simulink model "control_system"  (R2023a)
settings: Solver=VariableStepAuto  StartTime=0.0  StopTime=10.0  RelTol=1e-3
model workspace (MAT data in the model file):
  C_L = Simulink.Parameter
  C_L.Value = 1
  C_L.DataType = 'auto'
  C_L.Complexity = 'real'
  C_L.Dimensions = [1 1]
  C_R = Simulink.Parameter
  C_R.Value = 2
  C_R.DataType = 'auto'
  C_R.Complexity = 'real'
  C_R.Dimensions = [1 1]
  V = Simulink.Parameter
  V.Value = 1
  V.DataType = 'auto'
  V.DocUnits = 'm/s'
  V.Complexity = 'real'
  V.Dimensions = [1 1]
  b_w = Simulink.Parameter
  b_w.Value = 15
  b_w.DataType = 'auto'
  b_w.DocUnits = 'mm'
  b_w.Complexity = 'real'
  b_w.Dimensions = [1 1]
undefined symbols (not defined in the file): Ka
libraries: slpidlib x3
settings Model: Creator=gabrielle  LastModifiedBy=gabrielle

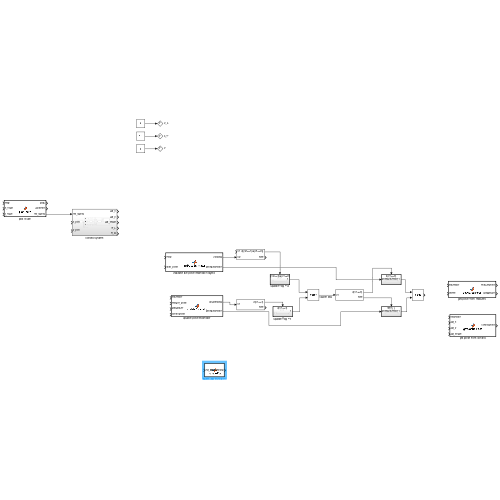
[thumbnail: Simulink's stored preview of the top-level diagram]
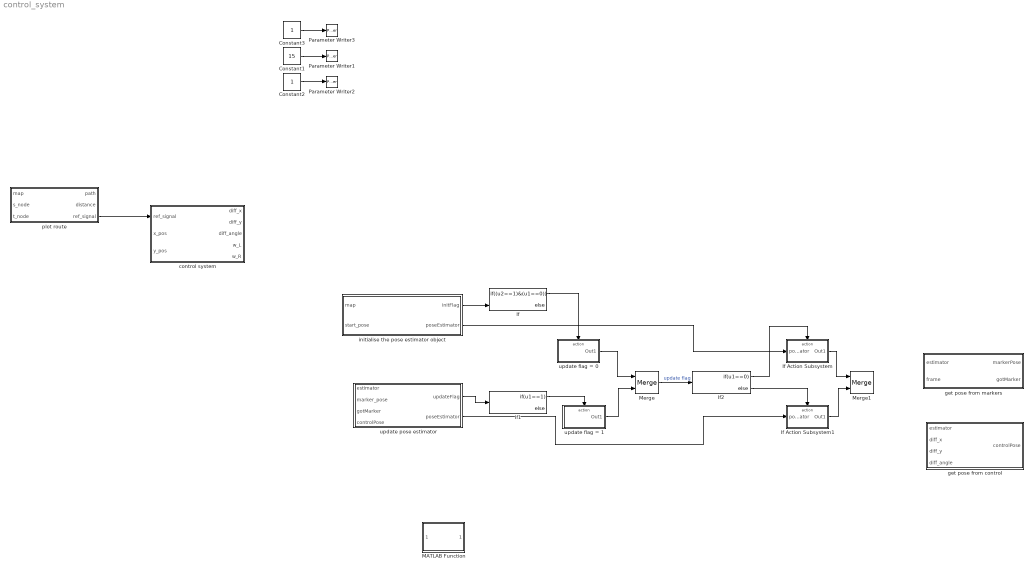
== system control_system ==
  Constant1 : Constant  Value=15
  Constant2 : Constant
  Constant3 : Constant
  If : If  NumInputs=2  IfExpression=(u2==1)&(u1==0)
  If Action Subsystem : Subsystem  TreatAsAtomicUnit=on
  If Action Subsystem1 : Subsystem  TreatAsAtomicUnit=on
  If1 : If  IfExpression=u1==1
  If2 : If  IfExpression=u1==0
  MATLAB Function : MATLAB Function  TreatAsAtomicUnit=on
  Merge : Merge  InitialOutput=0
  Merge1 : Merge  InitialOutput=0
  Parameter Writer1 : ParameterWriter  AccessWorkspaceVariable=on  WorkspaceVariableName=b_w
  Parameter Writer2 : ParameterWriter  AccessWorkspaceVariable=on  WorkspaceVariableName=V
  Parameter Writer3 : ParameterWriter  AccessWorkspaceVariable=on  WorkspaceVariableName=C_L
  control system : Subsystem
  get pose from control : MATLAB Function  TreatAsAtomicUnit=on
  get pose from markers : MATLAB Function  TreatAsAtomicUnit=on
  initialise the pose estimator object : MATLAB Function  TreatAsAtomicUnit=on
  plot route : MATLAB Function  TreatAsAtomicUnit=on
  update flag = 0 : Subsystem  TreatAsAtomicUnit=on
  update flag = 1 : Subsystem  TreatAsAtomicUnit=on
  update pose estimator : MATLAB Function  TreatAsAtomicUnit=on
  wires:
  Constant3/1 -> Parameter Writer3/1
  Constant1/1 -> Parameter Writer1/1
  Constant2/1 -> Parameter Writer2/1
  plot route/3(ref_signal) -> control system/1(ref_signal)
  initialise the pose estimator object/1(initFlag) -> If/2
  update pose estimator/1(updateFlag) -> If1/1
  update flag = 0/1(Out1) -> Merge/1
  update flag = 1/1(Out1) -> Merge/2
  If/1 -> update flag = 0/Action
  Merge/1 -> If2/1  "update flag"
  If1/1 -> update flag = 1/Action
  If2/1 -> If Action Subsystem/Action
  If2/2 -> If Action Subsystem1/Action
  initialise the pose estimator object/2(poseEstimator) -> If Action Subsystem/1(poseEstimator)
  update pose estimator/2(poseEstimator) -> If Action Subsystem1/1(poseEstimator)
  If Action Subsystem/1(Out1) -> Merge1/1
  If Action Subsystem1/1(Out1) -> Merge1/2

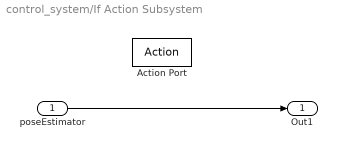
== system control_system/If Action Subsystem ==
  poseEstimator : Inport
  Action Port : ActionPort  ActionPortLabel=if(u1==0)
  Out1 : Outport
  wires:
  poseEstimator/1 -> Out1/1

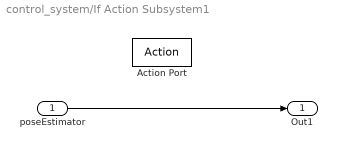
== system control_system/If Action Subsystem1 ==
  poseEstimator : Inport
  Action Port : ActionPort  ActionPortLabel=else
  Out1 : Outport
  wires:
  poseEstimator/1 -> Out1/1

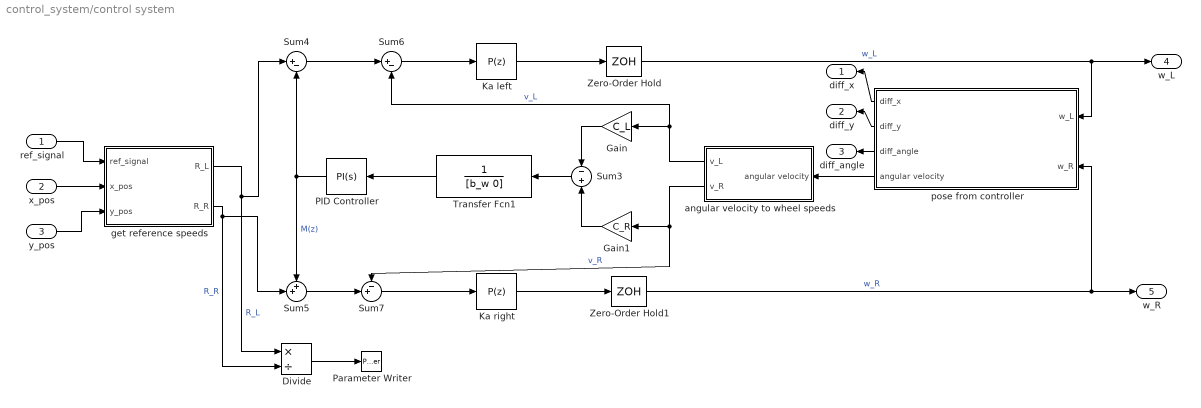
== system control_system/control system ==
  ref_signal : Inport
  x_pos : Inport  Port=2
  y_pos : Inport  Port=3
  Divide : Product  Inputs=*/
  Gain : Gain  Gain=C_L
  Gain1 : Gain  Gain=C_R
  Ka left : slpidlib/PID Controller  Controller=P  Form=Parallel  TimeDomain=Discrete-time  UseExternalTs=off  SampleTime=-1  IntegratorMethod=Forward Euler  FilterMethod=Forward Euler  ControllerParametersSource=internal  P=Ka  I=1  UseKiTs=off  D=0  N=100  UseFilter=on  TunerSelectOption=Transfer Function Based (PID Tuner App)  InitialConditionSource=internal  InitialConditionForIntegrator=0  InitialConditionForFilter=0  DifferentiatorICPrevScaledInput=0  ExternalReset=none  TrackingMode=off  Kt=1  LimitOutput=off  SatLimitsSource=internal  UpperSaturationLimit=inf  LowerSaturationLimit=-inf  LinearizeAsGain=off  AntiWindupMode=none  Kb=1  LimitIntegrator=off  UpperIntegratorSaturationLimit=inf  LowerIntegratorSaturationLimit=-inf  POutMin=[]  POutMax=[]  IOutMin=[]  IOutMax=[]  DOutMin=[]  DOutMax=[]  NOutMin=[]  NOutMax=[]  SumOutMin=[]  SumOutMax=[]  SaturationOutMin=[]  SaturationOutMax=[]  PParamMin=[]  PParamMax=[]  IParamMin=[]  IParamMax=[]  DParamMin=[]  DParamMax=[]  NParamMin=[]  NParamMax=[]  KbParamMin=[]  KbParamMax=[]  KtParamMin=[]  KtParamMax=[]  KbOutMin=[]  KbOutMax=[]  KtOutMin=[]  KtOutMax=[]  IntegratorOutMin=[]  IntegratorOutMax=[]  FilterOutMin=[]  FilterOutMax=[]  SumI1OutMin=[]  SumI1OutMax=[]  SumI2OutMin=[]  SumI2OutMax=[]  SumI3OutMin=[]  SumI3OutMax=[]  SumI4OutMin=[]  SumI4OutMax=[]  SumDOutMin=[]  SumDOutMax=[]  DifferentiatorOutMin=[]  DifferentiatorOutMax=[]  FilterDiffOutCoefMin=[]  FilterDiffOutCoefMax=[]  ReciprocalOutMin=[]  ReciprocalOutMax=[]  SumDenOutMin=[]  SumDenOutMax=[]  SumNumOutMin=[]  SumNumOutMax=[]  DivideOutMin=[]  DivideOutMax=[]  UdiffTsProdOutMin=[]  UdiffTsProdOutMax=[]  NTsProdOutMin=[]  NTsProdOutMax=[]  UintegralTsProdOutMin=[]  UintegralTsProdOutMax=[]  UngainTsProdOutMin=[]  UngainTsProdOutMax=[]  ClampingZeroOutDataTypeStr=Inherit: Inherit via back propagation  ClampingZeroOutMin=[]  ClampingZeroOutMax=[]  FilterDenConstantOutDataTypeStr=Inherit: Inherit via back propagation  FilterDenConstantOutMin=[]  FilterDenConstantOutMax=[]  PCopyOutDataTypeStr=Inherit: Inherit via back propagation  PCopyOutMin=[]  PCopyOutMax=[]  NCopyOutDataTypeStr=Inherit: Inherit via back propagation  NCopyOutMin=[]  NCopyOutMax=[]  IntegratorContinuousStateAttributes=''  IntegratorStateMustResolveToSignalObject=off  IntegratorRTWStateStorageClass=Auto  FilterContinuousStateAttributes=''  FilterStateMustResolveToSignalObject=off  FilterRTWStateStorageClass=Auto  ParallelPVariant=InternalParameters  IdealPVariant=Disabled  IVariant=Disabled  DVariant=Disabled  IntegratorVariant=Disabled  SatVariant=Disabled  AWVariant=Disabled  PCopyVariant=Disabled  TRVariant=Disabled  FdbkBlocksVariant=Forward  IdealPFdbkVariant=Disabled  SatFdbkVariant=Disabled  DerivativeFilterVariant=Disabled  NVariant=Disabled  NCopyVariant=Disabled_SignalSpec  FilterICVariant=Disabled  IntegratorICVariant=Disabled  ExternalResetVariant=Disabled  TRSumVariant=Passthrough  SumFdbkVariant=Disabled  SumVariant=Passthrough_P  TsampFilterVariant=InternalTs  TsampNgainVariant=Passthrough  TsampIntegralVariant=Disabled_SignalSpec  ExternalSaturationOutDataTypeStr=Inherit: Same as second input
      settings: LibrarySourceBlock=simulink/Discrete/Discrete PID Controller
  Ka right : slpidlib/PID Controller  Controller=P  Form=Parallel  TimeDomain=Discrete-time  UseExternalTs=off  SampleTime=-1  IntegratorMethod=Forward Euler  FilterMethod=Forward Euler  ControllerParametersSource=internal  P=Ka  I=1  UseKiTs=off  D=0  N=100  UseFilter=on  TunerSelectOption=Transfer Function Based (PID Tuner App)  InitialConditionSource=internal  InitialConditionForIntegrator=0  InitialConditionForFilter=0  DifferentiatorICPrevScaledInput=0  ExternalReset=none  TrackingMode=off  Kt=1  LimitOutput=off  SatLimitsSource=internal  UpperSaturationLimit=inf  LowerSaturationLimit=-inf  LinearizeAsGain=off  AntiWindupMode=none  Kb=1  LimitIntegrator=off  UpperIntegratorSaturationLimit=inf  LowerIntegratorSaturationLimit=-inf  POutMin=[]  POutMax=[]  IOutMin=[]  IOutMax=[]  DOutMin=[]  DOutMax=[]  NOutMin=[]  NOutMax=[]  SumOutMin=[]  SumOutMax=[]  SaturationOutMin=[]  SaturationOutMax=[]  PParamMin=[]  PParamMax=[]  IParamMin=[]  IParamMax=[]  DParamMin=[]  DParamMax=[]  NParamMin=[]  NParamMax=[]  KbParamMin=[]  KbParamMax=[]  KtParamMin=[]  KtParamMax=[]  KbOutMin=[]  KbOutMax=[]  KtOutMin=[]  KtOutMax=[]  IntegratorOutMin=[]  IntegratorOutMax=[]  FilterOutMin=[]  FilterOutMax=[]  SumI1OutMin=[]  SumI1OutMax=[]  SumI2OutMin=[]  SumI2OutMax=[]  SumI3OutMin=[]  SumI3OutMax=[]  SumI4OutMin=[]  SumI4OutMax=[]  SumDOutMin=[]  SumDOutMax=[]  DifferentiatorOutMin=[]  DifferentiatorOutMax=[]  FilterDiffOutCoefMin=[]  FilterDiffOutCoefMax=[]  ReciprocalOutMin=[]  ReciprocalOutMax=[]  SumDenOutMin=[]  SumDenOutMax=[]  SumNumOutMin=[]  SumNumOutMax=[]  DivideOutMin=[]  DivideOutMax=[]  UdiffTsProdOutMin=[]  UdiffTsProdOutMax=[]  NTsProdOutMin=[]  NTsProdOutMax=[]  UintegralTsProdOutMin=[]  UintegralTsProdOutMax=[]  UngainTsProdOutMin=[]  UngainTsProdOutMax=[]  ClampingZeroOutDataTypeStr=Inherit: Inherit via back propagation  ClampingZeroOutMin=[]  ClampingZeroOutMax=[]  FilterDenConstantOutDataTypeStr=Inherit: Inherit via back propagation  FilterDenConstantOutMin=[]  FilterDenConstantOutMax=[]  PCopyOutDataTypeStr=Inherit: Inherit via back propagation  PCopyOutMin=[]  PCopyOutMax=[]  NCopyOutDataTypeStr=Inherit: Inherit via back propagation  NCopyOutMin=[]  NCopyOutMax=[]  IntegratorContinuousStateAttributes=''  IntegratorStateMustResolveToSignalObject=off  IntegratorRTWStateStorageClass=Auto  FilterContinuousStateAttributes=''  FilterStateMustResolveToSignalObject=off  FilterRTWStateStorageClass=Auto  ParallelPVariant=InternalParameters  IdealPVariant=Disabled  IVariant=Disabled  DVariant=Disabled  IntegratorVariant=Disabled  SatVariant=Disabled  AWVariant=Disabled  PCopyVariant=Disabled  TRVariant=Disabled  FdbkBlocksVariant=Forward  IdealPFdbkVariant=Disabled  SatFdbkVariant=Disabled  DerivativeFilterVariant=Disabled  NVariant=Disabled  NCopyVariant=Disabled_SignalSpec  FilterICVariant=Disabled  IntegratorICVariant=Disabled  ExternalResetVariant=Disabled  TRSumVariant=Passthrough  SumFdbkVariant=Disabled  SumVariant=Passthrough_P  TsampFilterVariant=InternalTs  TsampNgainVariant=Passthrough  TsampIntegralVariant=Disabled_SignalSpec  ExternalSaturationOutDataTypeStr=Inherit: Same as second input
      settings: LibrarySourceBlock=simulink/Discrete/Discrete PID Controller
  PID Controller : slpidlib/PID Controller  Controller=PI  Form=Parallel  TimeDomain=Continuous-time  UseExternalTs=off  SampleTime=-1  IntegratorMethod=Forward Euler  FilterMethod=Forward Euler  ControllerParametersSource=internal  P=1  I=1  UseKiTs=off  D=0  N=100  UseFilter=on  TunerSelectOption=Transfer Function Based (PID Tuner App)  InitialConditionSource=internal  InitialConditionForIntegrator=0  InitialConditionForFilter=0  DifferentiatorICPrevScaledInput=0  ExternalReset=none  TrackingMode=off  Kt=1  LimitOutput=off  SatLimitsSource=internal  UpperSaturationLimit=inf  LowerSaturationLimit=-inf  LinearizeAsGain=on  AntiWindupMode=none  Kb=1  LimitIntegrator=off  UpperIntegratorSaturationLimit=inf  LowerIntegratorSaturationLimit=-inf  POutMin=[]  POutMax=[]  IOutMin=[]  IOutMax=[]  DOutMin=[]  DOutMax=[]  NOutMin=[]  NOutMax=[]  SumOutMin=[]  SumOutMax=[]  SaturationOutMin=[]  SaturationOutMax=[]  PParamMin=[]  PParamMax=[]  IParamMin=[]  IParamMax=[]  DParamMin=[]  DParamMax=[]  NParamMin=[]  NParamMax=[]  KbParamMin=[]  KbParamMax=[]  KtParamMin=[]  KtParamMax=[]  KbOutMin=[]  KbOutMax=[]  KtOutMin=[]  KtOutMax=[]  IntegratorOutMin=[]  IntegratorOutMax=[]  FilterOutMin=[]  FilterOutMax=[]  SumI1OutMin=[]  SumI1OutMax=[]  SumI2OutMin=[]  SumI2OutMax=[]  SumI3OutMin=[]  SumI3OutMax=[]  SumI4OutMin=[]  SumI4OutMax=[]  SumDOutMin=[]  SumDOutMax=[]  DifferentiatorOutMin=[]  DifferentiatorOutMax=[]  FilterDiffOutCoefMin=[]  FilterDiffOutCoefMax=[]  ReciprocalOutMin=[]  ReciprocalOutMax=[]  SumDenOutMin=[]  SumDenOutMax=[]  SumNumOutMin=[]  SumNumOutMax=[]  DivideOutMin=[]  DivideOutMax=[]  UdiffTsProdOutMin=[]  UdiffTsProdOutMax=[]  NTsProdOutMin=[]  NTsProdOutMax=[]  UintegralTsProdOutMin=[]  UintegralTsProdOutMax=[]  UngainTsProdOutMin=[]  UngainTsProdOutMax=[]  ClampingZeroOutDataTypeStr=Inherit: Inherit via back propagation  ClampingZeroOutMin=[]  ClampingZeroOutMax=[]  FilterDenConstantOutDataTypeStr=Inherit: Inherit via back propagation  FilterDenConstantOutMin=[]  FilterDenConstantOutMax=[]  PCopyOutDataTypeStr=Inherit: Inherit via back propagation  PCopyOutMin=[]  PCopyOutMax=[]  NCopyOutDataTypeStr=Inherit: Inherit via back propagation  NCopyOutMin=[]  NCopyOutMax=[]  IntegratorContinuousStateAttributes=''  IntegratorStateMustResolveToSignalObject=off  IntegratorRTWStateStorageClass=Auto  FilterContinuousStateAttributes=''  FilterStateMustResolveToSignalObject=off  FilterRTWStateStorageClass=Auto  ParallelPVariant=InternalParameters  IdealPVariant=Disabled  IVariant=InternalParameters  DVariant=Disabled  IntegratorVariant=Continuous  SatVariant=Disabled  AWVariant=Passthrough  PCopyVariant=Disabled  TRVariant=Disabled  FdbkBlocksVariant=Forward  IdealPFdbkVariant=Disabled  SatFdbkVariant=Disabled  DerivativeFilterVariant=Disabled  NVariant=Disabled  NCopyVariant=Disabled_SignalSpec  FilterICVariant=Disabled  IntegratorICVariant=InternalICs  ExternalResetVariant=Disabled  TRSumVariant=Passthrough  SumFdbkVariant=Disabled  SumVariant=Sum_PI  TsampFilterVariant=InternalTs  TsampNgainVariant=Passthrough  TsampIntegralVariant=Disabled_SignalSpec  ExternalSaturationOutDataTypeStr=Inherit: Same as second input
  Parameter Writer : ParameterWriter  AccessWorkspaceVariable=on  WorkspaceVariableName=C_R
  Sum3 : Sum  Inputs=-|+
  Sum4 : Sum  Inputs=|+-
  Sum5 : Sum  Inputs=++|
  Sum6 : Sum  Inputs=|+-
  Sum7 : Sum  Inputs=-+|
  Transfer Fcn1 : TransferFcn  Denominator=[b_w 0]
  Zero-Order Hold : ZeroOrderHold  SampleTime=-1
  Zero-Order Hold1 : ZeroOrderHold  SampleTime=-1
  angular velocity to wheel speeds : Subsystem
  get reference speeds : Subsystem
  pose from controller : Subsystem
  diff_x : Outport
  diff_y : Outport  Port=2
  diff_angle : Outport  Port=3
  w_L : Outport  Port=4
  w_R : Outport  Port=5
  wires:
  pose from controller/1(diff_x) -> diff_x/1
  Zero-Order Hold1/1 -> w_R/1, pose from controller/2(w_R)  "w_R"
  get reference speeds/1(R_L) -> Divide/1, Sum4/1  "R_L"
  pose from controller/4(angular velocity) -> angular velocity to wheel speeds/1(angular velocity)
  Sum5/1 -> Sum7/2
  Sum4/1 -> Sum6/1
  angular velocity to wheel speeds/2(v_R) -> Sum7/1, Gain1/1  "v_R"
  get reference speeds/2(R_R) -> Sum5/2, Divide/2  "R_R"
  Zero-Order Hold/1 -> w_L/1, pose from controller/1(w_L)  "w_L"
  x_pos/1 -> get reference speeds/2(x_pos)
  Divide/1 -> Parameter Writer/1
  angular velocity to wheel speeds/1(v_L) -> Sum6/2, Gain/1  "v_L"
  ref_signal/1 -> get reference speeds/1(ref_signal)
  pose from controller/3(diff_angle) -> diff_angle/1
  PID Controller/1 -> Sum5/1, Sum4/2  "M(z)"
  Ka right/1 -> Zero-Order Hold1/1
  Sum6/1 -> Ka left/1
  y_pos/1 -> get reference speeds/3(y_pos)
  Sum7/1 -> Ka right/1
  Transfer Fcn1/1 -> PID Controller/1
  Ka left/1 -> Zero-Order Hold/1
  Gain/1 -> Sum3/1
  Sum3/1 -> Transfer Fcn1/1
  pose from controller/2(diff_y) -> diff_y/1
  Gain1/1 -> Sum3/2

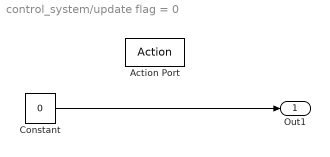
== system control_system/update flag = 0 ==
  Action Port : ActionPort  ActionPortLabel=if((u2==1)&(u1==0))
  Constant : Constant  Value=0
  Out1 : Outport
  wires:
  Constant/1 -> Out1/1

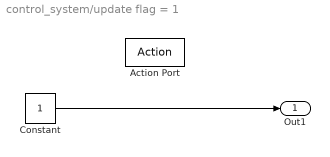
== system control_system/update flag = 1 ==
  Action Port : ActionPort  ActionPortLabel=if(u1==1)
  Constant : Constant
  Out1 : Outport
  wires:
  Constant/1 -> Out1/1

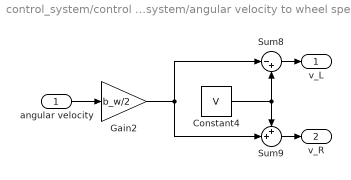
== system control_system/control system/angular velocity to wheel speeds ==
  angular velocity : Inport
  Constant4 : Constant  Value=V  VectorParams1D=off
  Gain2 : Gain  Gain=b_w/2
  Sum8 : Sum  Inputs=|-+
  Sum9 : Sum  Inputs=++|
  v_L : Outport
  v_R : Outport  Port=2
  wires:
  Sum9/1 -> v_R/1
  angular velocity/1 -> Gain2/1
  Sum8/1 -> v_L/1
  Gain2/1 -> Sum9/2, Sum8/1
  Constant4/1 -> Sum9/1, Sum8/2

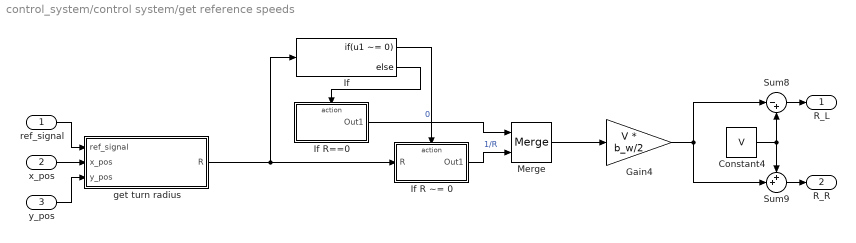
== system control_system/control system/get reference speeds ==
  ref_signal : Inport
  x_pos : Inport  Port=2
  y_pos : Inport  Port=3
  Constant4 : Constant  Value=V
  Gain4 : Gain  Gain=V * b_w/2
  If : If  IfExpression=u1 ~= 0
  If R ~= 0 : Subsystem  TreatAsAtomicUnit=on
  If R==0 : Subsystem  TreatAsAtomicUnit=on
  Merge : Merge  InitialOutput=0
  Sum8 : Sum  Inputs=|-+
  Sum9 : Sum  Inputs=++|
  get turn radius : MATLAB Function  TreatAsAtomicUnit=on
  R_L : Outport
  R_R : Outport  Port=2
  wires:
  x_pos/1 -> get turn radius/2(x_pos)
  y_pos/1 -> get turn radius/3(y_pos)
  Merge/1 -> Gain4/1
  Sum9/1 -> R_R/1
  Gain4/1 -> Sum9/2, Sum8/1
  If/1 -> If R ~= 0/Action
  If/2 -> If R==0/Action
  If R==0/1(Out1) -> Merge/1  "0"
  Constant4/1 -> Sum9/1, Sum8/2
  If R ~= 0/1(Out1) -> Merge/2  "1/R"
  Sum8/1 -> R_L/1
  get turn radius/1(R) -> If/1, If R ~= 0/1(R)
  ref_signal/1 -> get turn radius/1(ref_signal)

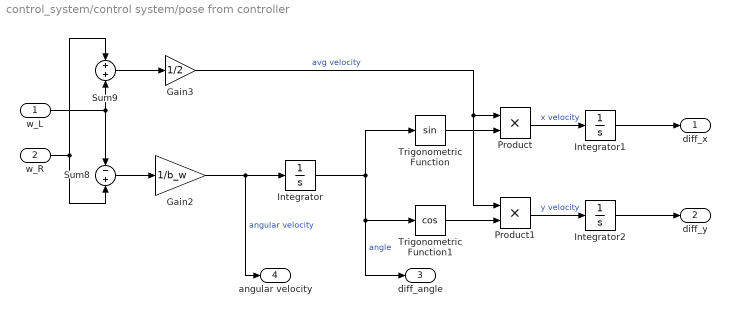
== system control_system/control system/pose from controller ==
  w_L : Inport
  w_R : Inport  Port=2
  Gain2 : Gain  Gain=1/b_w
  Gain3 : Gain  Gain=1/2
  Integrator : Integrator
  Integrator1 : Integrator
  Integrator2 : Integrator
  Product : Product
  Product1 : Product
  Sum8 : Sum  Inputs=-|+
  Sum9 : Sum  Inputs=+|+
  Trigonometric Function : Trigonometry
  Trigonometric Function1 : Trigonometry  Operator=cos
  diff_x : Outport
  diff_y : Outport  Port=2
  diff_angle : Outport  Port=3
  angular velocity : Outport  Port=4
  wires:
  Integrator2/1 -> diff_y/1
  Product/1 -> Integrator1/1  "x velocity"
  Sum9/1 -> Gain3/1
  Integrator1/1 -> diff_x/1
  Product1/1 -> Integrator2/1  "y velocity"
  w_R/1 -> Sum8/2, Sum9/1
  Trigonometric Function1/1 -> Product1/2
  Gain3/1 -> Product/1, Product1/1  "avg velocity"
  Trigonometric Function/1 -> Product/2
  Integrator/1 -> diff_angle/1, Trigonometric Function1/1, Trigonometric Function/1  "angle"
  Gain2/1 -> angular velocity/1, Integrator/1  "angular velocity"
  w_L/1 -> Sum8/1, Sum9/2
  Sum8/1 -> Gain2/1

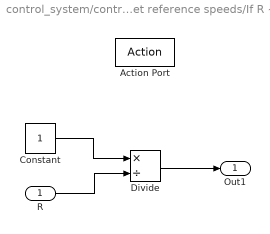
== system control_system/control system/get reference speeds/If R ~= 0 ==
  R : Inport
  Action Port : ActionPort  ActionPortLabel=if(u1 ~= 0)
  Constant : Constant
  Divide : Product  Inputs=*/
  Out1 : Outport
  wires:
  Constant/1 -> Divide/1
  R/1 -> Divide/2
  Divide/1 -> Out1/1

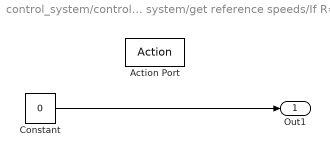
== system control_system/control system/get reference speeds/If R==0 ==
  Action Port : ActionPort  ActionPortLabel=else
  Constant : Constant  Value=0
  Out1 : Outport
  wires:
  Constant/1 -> Out1/1

== matlab function control_system/plot route ==
  data: path output; distance output; ref_signal output; map input; s_node input; t_node input
function [path, distance, ref_signal] = plotRoute(map, s_node, t_node)
% plotRoute     plot the route from the start node to the stop node
% Inputs:
%   map     : current map object
%   s_node  : starting node object
%   t_node  : stop node object
% Outputs:
%   path        : shortest path between the two nodes - array of node IDs
%   distance    : total distance of path
%   ref_signal  : reference signal for the path - cell array of
%                   path_segment objects
%
% See also map, node, path_segment

routePlanner = route_planner(map);
[path, distance] = plot_route(routePlanner, s_node, t_node);

ref_signal = convert_to_ref(routePlanner, path);

== matlab function control_system/control system/get reference speeds/get turn radius ==
  data: ref_signal input; R output; x_pos input; y_pos input
function R = getRadius(ref_signal, x_pos, y_pos)
% getRadius     get the turn radius of the current path segment
% Inputs:
%   ref_signal  : reference signal - cell array of path_segments
%   x_pos       : estimated x coordinate
%   y_pos       : estimated y coordinate
%
% Outputs:
%   R   : turn radius of current path segment
%
% See also path_segment

persistent n

if isempty(n)
    n = 1;
end

segment = ref_signal{n};
R = segment.R;

x_check = (x_pos <= segment.stop(1)*0.9) && (x_pos >= segment.stop(1)*1.1); % x_pos within 10% of stop node x coord
y_check = (y_pos <= segment.stop(2)*0.9) && (y_pos >= segment.stop(2)*1.1); % y_pos within 10% of stop node y coord

if x_check && y_check
    n = n+1;
end

== matlab function control_system/initialise the pose estimator object ==
  data: initFlag output; poseEstimator output; map input; start_pose input
function [initFlag, poseEstimator] = initPoseEstimator(map, start_pose)
poseEstimator = pose_estimator(map, start_pose);
initFlag = 0;

== matlab function control_system/get pose from markers ==
  data: estimator input; markerPose output; frame input; gotMarker output
function [markerPose, gotMarker] = getMarkerPose(estimator, frame)
if ~isempty(frame)
    [id, loc, pose] = find_markers(estimator, frame);
    markerPose = pose_from_marker(estimator, loc, pose);
    gotMarker = 1;
else
    markerPose = [404; 404; 404];
    gotMarker = 0;
end

== matlab function control_system/get pose from control ==
  data: controlPose output; estimator input; diff_x input; diff_y input; diff_angle input
function controlPose = getControlPose(estimator, diff_x, diff_y, diff_angle)
controlPose = pose_from_control(estimator, diff_x, diff_y, diff_angle);

== matlab function control_system/update pose estimator ==
  data: updateFlag output; estimator input; poseEstimator output; marker_pose input; gotMarker input; controlPose input
function [updateFlag, poseEstimator] = updateEstimator(estimator, marker_pose, gotMarker, controlPose)
poseEstimator = update_pose(estimator, marker_pose, gotMarker, controlPose);
updateFlag = 1;

== matlab function control_system/MATLAB Function ==
  data: init_flag input; updateFlag output
function updateFlag = manageFlag(init_flag)
persistent flag

if (isempty(flag)&&(init_flag == 1))
    flag = 0;
elseif (flag == 0)
    flag = 1;
end

updateFlag = flag;
